simulink model "gm_sampleModel1533_sub"  (R2023a)
settings: Solver=VariableStepAuto  StartTime=0.0  StopTime=10.0  RelTol=1e-3
libraries: simulink x1
settings Model: Creator=user1  LastModifiedBy=user1
settings OptimizationCC: BlockReduction=off  ConditionallyExecuteInputs=off
settings DebuggingCC: InheritedTsInSrcMsg=none

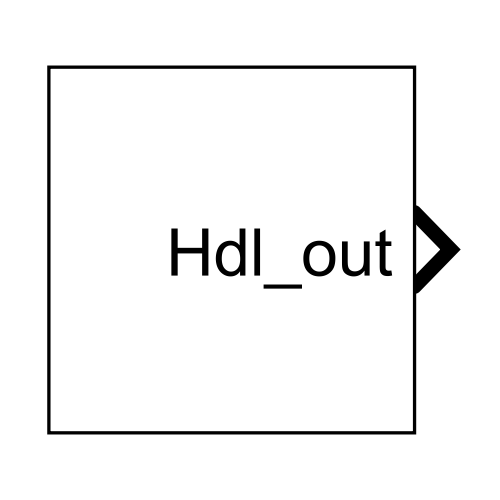
[thumbnail: Simulink's stored preview of the top-level diagram]
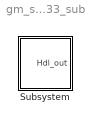
== system gm_sampleModel1533_sub ==
  Subsystem : Subsystem

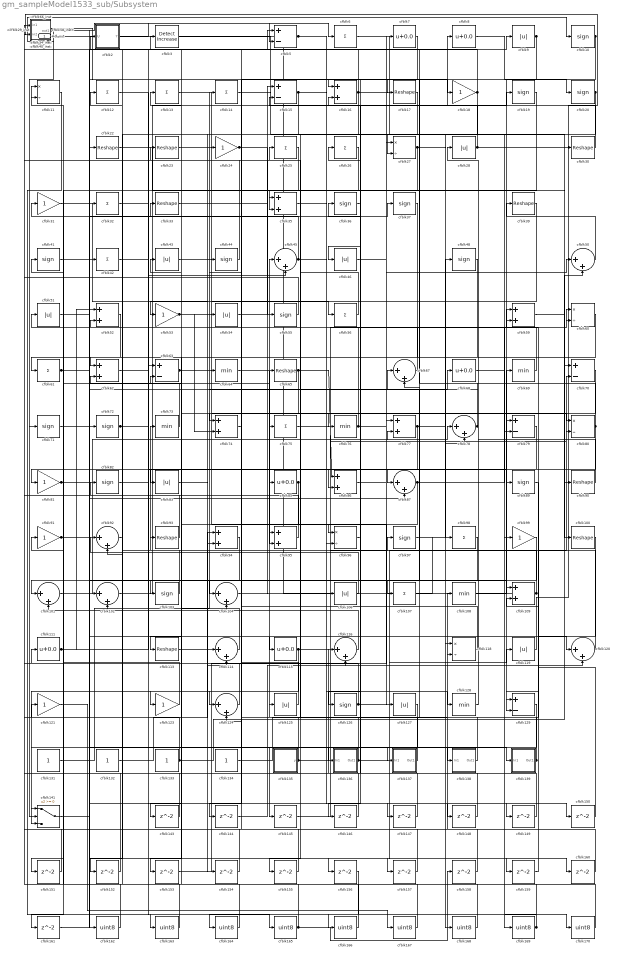
== system gm_sampleModel1533_sub/Subsystem ==
  cfblk1 : Constant  Value=0  OutDataTypeStr=uint8  SampleTime=1
  cfblk{10,19..20,36..37,41,44,48,55,71..72,82,89,97,103,126} (16 alike) : Signum
  cfblk{17,22..23,30,33,39,65,90,93,100,113} (11 alike) : Reshape
  cfblk{45,50,67,78,87,92,101..102,104,114,116,120,124} (13 alike) : Sum  Inputs=|++  OutDataTypeStr=uint8
  cfblk105_inst : Subsystem
  cfblk{9,28,43,46,51,54,83,106,119,125,127} (11 alike) : Abs  OutDataTypeStr=uint8  SaturateOnIntegerOverflow=off
  cfblk{6,12..14,25..26,32,42,56,61,75,98,107} (13 alike) : Sum  Inputs=+  OutDataTypeStr=uint8
  cfblk{64,69,73,76,108,128} (6 alike) : MinMax  OutDataTypeStr=uint8
  cfblk{16,35,52,59,62,74,77,86,94..95,109} (11 alike) : Sum  OutDataTypeStr=uint8
  cfblk{11,27,60,80,96,118} (6 alike) : Product  Inputs=*/  OutDataTypeStr=uint8  RndMeth=Zero  SaturateOnIntegerOverflow=on
  cfblk110_inst : Subsystem
  cfblk{7..8,68,85,111,115} (6 alike) : Bias  Bias=0.0  SaturateOnIntegerOverflow=off
  cfblk112_inst : Subsystem
  cfblk117_inst : Subsystem
  cfblk{18,24,31,53,81,91,99,121,123} (9 alike) : Gain  OutDataTypeStr=uint8
  cfblk122_inst : Subsystem
  cfblk{5,15,63,70,79,129} (6 alike) : Sum  Inputs=+-  OutDataTypeStr=uint8
  cfblk{131..134} (4 alike) : Constant  OutDataTypeStr=uint8  SampleTime=-1
  cfblk135 : Subsystem  mask(Counter Free-Running){NumBits=double(16), tsamp=double(-1)}
      mask prompts: NumBits "Simulink:masks:NumberOfBits_MP"; tsamp "Simulink:masks:SampleTime_MP"
      mask help: Simulink:masks:CounterFreeRunning_MD
  cfblk136 : Subsystem
  cfblk137 : Subsystem
  cfblk138 : Subsystem
  cfblk139 : Subsystem
  cfblk141 : Switch  OutDataTypeStr=uint8  SaturateOnIntegerOverflow=off  InputSameDT=off
  cfblk{143..161} (19 alike) : Delay  SampleTime=1
  cfblk{162..170} (9 alike) : DataTypeConversion  OutDataTypeStr=uint8  SaturateOnIntegerOverflow=off  RndMeth=Floor
  cfblk2 : Subsystem  mask(Detect Rise Nonnegative){vinit=double(0), InputProcessing=Elements as channels (sample based), OutDataTypeStr=uint8}
      mask prompts: vinit "Simulink:masks:InitialCondition_MP"; InputProcessing "Simulink:masks:InputProcessing_MP"; OutDataTypeStr "Simulink:masks:OutputDataType_MP"
      mask help: Simulink:masks:DetectRiseNonnegative_MD
      mask init:
      | InputProcessing = 'Elements as channels (sample based)';
      | OutDataTypeStr = 'uint8';
      | vinit = double(0);
      mask TypeOptions InputProcessing: Simulink:masks:ColumnsAsChannelsFrameBased | Simulink:masks:ElementsAsChannelsSampleBased
      mask TypeOptions OutDataTypeStr: Simulink:masks:uint8 | Simulink:masks:boolean
      mask Display: fprintf('U >= 0\n&  NOT\nU/z >= 0')
  cfblk21_inst : Subsystem
  cfblk29_inst : Subsystem
  cfblk3 : simulink/Logic and Bit Operations/Detect Increase  vinit=0.0  OutDataTypeStr=uint8
      settings: LibrarySourceBlock=|
      | hdlsllib/Logic and Bit
      | Operations/Detect
      | Increase
  cfblk34_inst : Subsystem
  cfblk40_inst : Subsystem
  cfblk58_inst : Subsystem
  cfblk66_inst : Subsystem
  Hdl_out : Outport  OutDataTypeStr=uint8  SampleTime=1
  wires:
  cfblk1/1 -> cfblk16/1
  cfblk10/1 -> cfblk67/2, cfblk46/1, cfblk129/2
  cfblk100/1 -> cfblk111/1
  cfblk101/1 -> cfblk78/1
  cfblk102/1 -> cfblk19/1
  cfblk103/1 -> cfblk73/1
  cfblk104/1 -> cfblk97/1
  cfblk105_inst/1(out1) -> cfblk10/1
  cfblk106/1 -> cfblk92/1
  cfblk107/1 -> cfblk98/1
  cfblk108/1 -> cfblk69/1
  cfblk109/1 -> Hdl_out/1, cfblk2/1(U)
  cfblk11/1 -> cfblk163/1
  cfblk110_inst/1(out1) -> cfblk22/1, cfblk160/1
  cfblk111/1 -> cfblk63/1, cfblk52/1
  cfblk112_inst/1(out1) -> cfblk109/1
  cfblk113/1 -> cfblk114/1
  cfblk114/1 -> cfblk13/1
  cfblk115/1 -> cfblk79/1, cfblk77/2, cfblk141/3
  cfblk116/1 -> cfblk101/2
  cfblk117_inst/1(out1) -> cfblk103/1
  cfblk118/1 -> cfblk33/1
  cfblk119/1 -> cfblk66_inst/2(in2)
  cfblk12/1 -> cfblk45/2
  cfblk120/1 -> cfblk59/1
  cfblk121/1 -> cfblk167/1
  cfblk122_inst/1(out1) -> cfblk162/1
  cfblk123/1 -> cfblk91/1
  cfblk124/1 -> cfblk21_inst/2(in2)
  cfblk125/1 -> cfblk93/1
  cfblk126/1 -> cfblk70/2, cfblk43/1
  cfblk127/1 -> cfblk141/1
  cfblk128/1 -> cfblk28/1
  cfblk129/1 -> cfblk145/1
  cfblk13/1 -> cfblk56/1
  cfblk131/1 -> cfblk14/1
  cfblk132/1 -> cfblk94/1
  cfblk133/1 -> cfblk62/2, cfblk50/2, cfblk112_inst/2(in2)
  cfblk134/1 -> cfblk108/1
  cfblk135/1(y) -> cfblk52/2, cfblk60/1
  cfblk136/1(Out1) -> cfblk45/1, cfblk119/1, cfblk159/1, cfblk25/1
  cfblk137/1(Out1) -> cfblk40_inst/1(in1)
  cfblk138/1(Out1) -> cfblk125/1
  cfblk139/1(Out1) -> cfblk67/1, cfblk36/1
  cfblk14/1 -> cfblk70/1
  cfblk141/1 -> cfblk72/1
  cfblk143/1 -> cfblk11/1
  cfblk144/1 -> cfblk120/2
  cfblk145/1 -> cfblk80/2
  cfblk146/1 -> cfblk105_inst/1(in1)
  cfblk147/1 -> cfblk16/2
  cfblk148/1 -> cfblk40_inst/2(in2)
  cfblk149/1 -> cfblk116/1
  cfblk15/1 -> cfblk92/2, cfblk27/2
  cfblk150/1 -> cfblk59/2
  cfblk151/1 -> cfblk117_inst/2(in2)
  cfblk152/1 -> cfblk110_inst/1(in1)
  cfblk153/1 -> cfblk77/1
  cfblk154/1 -> cfblk21_inst/1(in1)
  cfblk155/1 -> cfblk63/2
  cfblk156/1 -> cfblk164/1
  cfblk157/1 -> cfblk104/2
  cfblk158/1 -> cfblk58_inst/1(in1)
  cfblk159/1 -> cfblk109/2
  cfblk16/1 -> cfblk95/2, cfblk78/2, cfblk112_inst/1(in1)
  cfblk160/1 -> cfblk118/2
  cfblk161/1 -> cfblk9/1
  cfblk162/1 -> cfblk58_inst/2(in2)
  cfblk163/1 -> cfblk122_inst/1(in1)
  cfblk164/1 -> cfblk122_inst/2(in2)
  cfblk165/1 -> cfblk158/1, cfblk12/1
  cfblk166/1 -> cfblk82/1
  cfblk167/1 -> cfblk34_inst/1(in1)
  cfblk168/1 -> cfblk121/1
  cfblk169/1 -> cfblk34_inst/2(in2), cfblk166/1
  cfblk17/1 -> cfblk94/2
  cfblk170/1 -> cfblk3/1
  cfblk18/1 -> cfblk66_inst/1(in1), cfblk62/1
  cfblk19/1 -> cfblk35/2
  cfblk2/1(Y) -> cfblk6/1
  cfblk20/1 -> cfblk87/1, cfblk124/2
  cfblk21_inst/1(out1) -> cfblk71/1, cfblk156/1
  cfblk22/1 -> cfblk100/1
  cfblk23/1 -> cfblk127/1
  cfblk24/1 -> cfblk106/1, cfblk96/1
  cfblk25/1 -> cfblk81/1
  cfblk26/1 -> cfblk35/1
  cfblk27/1 -> cfblk168/1, cfblk146/1
  cfblk28/1 -> cfblk8/1, cfblk30/1
  cfblk29_inst/1(out1) -> cfblk141/2, cfblk18/1
  cfblk3/1 -> cfblk169/1
  cfblk30/1 -> cfblk15/2
  cfblk31/1 -> cfblk114/2
  cfblk32/1 -> cfblk136/1(In1)
  cfblk33/1 -> cfblk55/1
  cfblk34_inst/1(out1) -> cfblk5/2, cfblk116/2
  cfblk35/1 -> cfblk79/2
  cfblk36/1 -> cfblk126/1
  cfblk37/1 -> cfblk101/1
  cfblk39/1 -> cfblk53/1
  cfblk40_inst/1(out1) -> cfblk42/1
  cfblk41/1 -> cfblk32/1
  cfblk42/1 -> cfblk138/1(In1)
  cfblk43/1 -> cfblk96/2
  cfblk44/1 -> cfblk29_inst/1(in1)
  cfblk45/1 -> cfblk31/1, cfblk128/1
  cfblk46/1 -> cfblk27/1
  cfblk48/1 -> cfblk123/1
  cfblk5/1 -> cfblk148/1, cfblk147/1
  cfblk50/1 -> cfblk39/1
  cfblk51/1 -> cfblk150/1
  cfblk52/1 -> cfblk61/1
  cfblk53/1 -> cfblk89/1, cfblk74/2
  cfblk54/1 -> cfblk15/1
  cfblk55/1 -> cfblk117_inst/1(in1)
  cfblk56/1 -> cfblk23/1
  cfblk58_inst/1(out1) -> cfblk120/1
  cfblk59/1 -> cfblk90/1
  cfblk6/1 -> cfblk118/1
  cfblk60/1 -> cfblk83/1
  cfblk61/1 -> cfblk115/1, cfblk137/1(In1)
  cfblk62/1 -> cfblk86/2
  cfblk63/1 -> cfblk95/1, cfblk99/1
  cfblk64/1 -> cfblk75/1
  cfblk65/1 -> cfblk86/1, cfblk104/1
  cfblk66_inst/1(out1) -> cfblk102/1
  cfblk67/1 -> cfblk54/1
  cfblk68/1 -> cfblk170/1
  cfblk69/1 -> cfblk44/1
  cfblk7/1 -> cfblk17/1
  cfblk70/1 -> cfblk153/1
  cfblk71/1 -> cfblk87/2
  cfblk72/1 -> cfblk5/1, cfblk149/1
  cfblk73/1 -> cfblk11/2
  cfblk74/1 -> cfblk24/1
  cfblk75/1 -> cfblk80/1
  cfblk76/1 -> cfblk7/1, cfblk51/1
  cfblk77/1 -> cfblk102/2, cfblk139/1(In1)
  cfblk78/1 -> cfblk29_inst/2(in2), cfblk76/1
  cfblk79/1 -> cfblk151/1
  cfblk8/1 -> cfblk20/1
  cfblk80/1 -> cfblk85/1, cfblk110_inst/2(in2)
  cfblk81/1 -> cfblk68/1, cfblk65/1
  cfblk82/1 -> cfblk165/1
  cfblk83/1 -> cfblk154/1
  cfblk85/1 -> cfblk144/1, cfblk143/1
  cfblk86/1 -> cfblk50/1
  cfblk87/1 -> cfblk60/2, cfblk155/1
  cfblk89/1 -> cfblk129/1
  cfblk9/1 -> cfblk74/1, cfblk107/1
  cfblk90/1 -> cfblk64/1
  cfblk91/1 -> cfblk37/1, cfblk157/1
  cfblk92/1 -> cfblk152/1
  cfblk93/1 -> cfblk105_inst/2(in2)
  cfblk94/1 -> cfblk113/1
  cfblk95/1 -> cfblk41/1
  cfblk96/1 -> cfblk26/1
  cfblk97/1 -> cfblk48/1
  cfblk98/1 -> cfblk161/1
  cfblk99/1 -> cfblk124/1

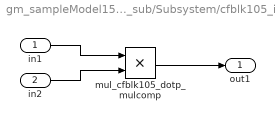
== system gm_sampleModel1533_sub/Subsystem/cfblk105_inst ==
  in1 : Inport  OutDataTypeStr=uint8  SampleTime=1
  in2 : Inport  Port=2  OutDataTypeStr=uint8  SampleTime=1
  mul_cfblk105_dotp_mulcomp : Product  Inputs=**  OutDataTypeStr=uint8  SampleTime=1
  out1 : Outport  OutDataTypeStr=uint8  SampleTime=1
  wires:
  in1/1 -> mul_cfblk105_dotp_mulcomp/1
  in2/1 -> mul_cfblk105_dotp_mulcomp/2
  mul_cfblk105_dotp_mulcomp/1 -> out1/1

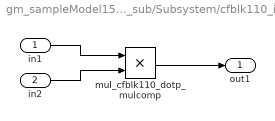
== system gm_sampleModel1533_sub/Subsystem/cfblk110_inst ==
  in1 : Inport  OutDataTypeStr=uint8  SampleTime=1
  in2 : Inport  Port=2  OutDataTypeStr=uint8  SampleTime=1
  mul_cfblk110_dotp_mulcomp : Product  Inputs=**  OutDataTypeStr=uint8  SampleTime=1
  out1 : Outport  OutDataTypeStr=uint8  SampleTime=1
  wires:
  in1/1 -> mul_cfblk110_dotp_mulcomp/1
  in2/1 -> mul_cfblk110_dotp_mulcomp/2
  mul_cfblk110_dotp_mulcomp/1 -> out1/1

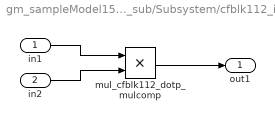
== system gm_sampleModel1533_sub/Subsystem/cfblk112_inst ==
  in1 : Inport  OutDataTypeStr=uint8  SampleTime=1
  in2 : Inport  Port=2  OutDataTypeStr=uint8  SampleTime=1
  mul_cfblk112_dotp_mulcomp : Product  Inputs=**  OutDataTypeStr=uint8  SampleTime=1
  out1 : Outport  OutDataTypeStr=uint8  SampleTime=1
  wires:
  in1/1 -> mul_cfblk112_dotp_mulcomp/1
  in2/1 -> mul_cfblk112_dotp_mulcomp/2
  mul_cfblk112_dotp_mulcomp/1 -> out1/1

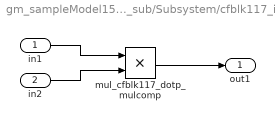
== system gm_sampleModel1533_sub/Subsystem/cfblk117_inst ==
  in1 : Inport  OutDataTypeStr=uint8  SampleTime=1
  in2 : Inport  Port=2  OutDataTypeStr=uint8  SampleTime=1
  mul_cfblk117_dotp_mulcomp : Product  Inputs=**  OutDataTypeStr=uint8  SampleTime=1
  out1 : Outport  OutDataTypeStr=uint8  SampleTime=1
  wires:
  in1/1 -> mul_cfblk117_dotp_mulcomp/1
  in2/1 -> mul_cfblk117_dotp_mulcomp/2
  mul_cfblk117_dotp_mulcomp/1 -> out1/1

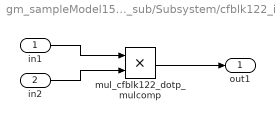
== system gm_sampleModel1533_sub/Subsystem/cfblk122_inst ==
  in1 : Inport  OutDataTypeStr=uint8  SampleTime=1
  in2 : Inport  Port=2  OutDataTypeStr=uint8  SampleTime=1
  mul_cfblk122_dotp_mulcomp : Product  Inputs=**  OutDataTypeStr=uint8  SampleTime=1
  out1 : Outport  OutDataTypeStr=uint8  SampleTime=1
  wires:
  in1/1 -> mul_cfblk122_dotp_mulcomp/1
  in2/1 -> mul_cfblk122_dotp_mulcomp/2
  mul_cfblk122_dotp_mulcomp/1 -> out1/1

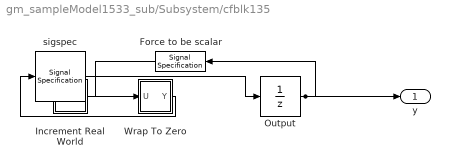
== system gm_sampleModel1533_sub/Subsystem/cfblk135 ==
  Force to be scalar : SignalSpecification  DisableCoverage=on  Dimensions=1
  Increment Real World : Subsystem  mask(Real World Value Increment){}
      mask help: Simulink:masks:RealWorldValueIncrement_MD
      mask Display: disp('V++')
  Output : UnitDelay  InitialCondition=0.0  SampleTime=tsamp  HasFrameUpgradeWarning=on
  Wrap To Zero : Subsystem  mask(Wrap To Zero){Threshold=double(65535)}
      mask prompts: Threshold "Simulink:masks:Threshold_MP"
      mask help: Simulink:masks:WrapToZero_MD
  sigspec : SignalSpecification  OutDataTypeStr=uint16  Dimensions=1
  y : Outport  SampleTime=1
  wires:
  Force to be scalar/1 -> Increment Real World/1(u)
  Increment Real World/1(y) -> Wrap To Zero/1(U)
  Output/1 -> Force to be scalar/1, y/1
  Wrap To Zero/1(Y) -> sigspec/1
  sigspec/1 -> Output/1

== system gm_sampleModel1533_sub/Subsystem/cfblk136 ==
  In1 : Inport  OutDataTypeStr=uint8  PortDimensions=1  SampleTime=1
  Out1 : Outport  SampleTime=1
  wires:
  In1/1 -> Out1/1

== system gm_sampleModel1533_sub/Subsystem/cfblk137 ==
  In1 : Inport  OutDataTypeStr=uint8  PortDimensions=1  SampleTime=1
  Out1 : Outport  SampleTime=1
  wires:
  In1/1 -> Out1/1

== system gm_sampleModel1533_sub/Subsystem/cfblk138 ==
  In1 : Inport  OutDataTypeStr=uint8  PortDimensions=1  SampleTime=1
  Out1 : Outport  SampleTime=1
  wires:
  In1/1 -> Out1/1

== system gm_sampleModel1533_sub/Subsystem/cfblk139 ==
  In1 : Inport  OutDataTypeStr=uint8  PortDimensions=1  SampleTime=1
  Out1 : Outport  SampleTime=1
  wires:
  In1/1 -> Out1/1

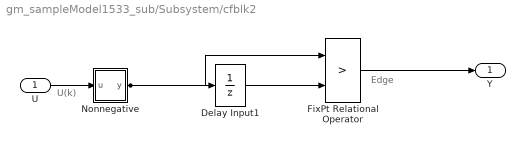
== system gm_sampleModel1533_sub/Subsystem/cfblk2 ==
  note: U(k)
  note: Edge
  U : Inport  OutDataTypeStr=uint8  SampleTime=1
  Delay Input1 : UnitDelay  Description=Store in Global RAM  DisableCoverage=on  InitialCondition=vinit  SampleTime=-1  HasFrameUpgradeWarning=on
  FixPt Relational Operator : RelationalOperator  Operator=>  OutDataTypeStr=fixdt(0, 8)  ZeroCross=off  InputSameDT=off
  Nonnegative : Subsystem  mask(Compare To Zero){relop=>=, OutDataTypeStr=boolean, ZeroCross=off}
      mask prompts: relop "Simulink:masks:Operator_MP"; OutDataTypeStr "Simulink:masks:OutputDataType_MP"; ZeroCross "Simulink:masks:EnableZerocrossingDetection_MP"
      mask help: Simulink:masks:CompareToZero_MD
      mask init:
      | OutDataTypeStr = 'boolean';
      | ZeroCross = 'off';
      | blkName = 'sampleModel1533_sub/Subsystem/cfblk2/Nonnegative';
      | relop = '>=';
      | setValue = 'boolean';
      mask TypeOptions relop: == | ~= | < | <= | >= | >
      mask TypeOptions OutDataTypeStr: Simulink:masks:uint8 | Simulink:masks:boolean
      mask Callback ZeroCross: sl('zeroCrossEnable', gcbh);
      mask Display: disp([relop,' 0'])
  Y : Outport  SampleTime=1
  wires:
  U/1 -> Nonnegative/1(u)
  Delay Input1/1 -> FixPt Relational Operator/2
  FixPt Relational Operator/1 -> Y/1
  Nonnegative/1(y) -> FixPt Relational Operator/1, Delay Input1/1

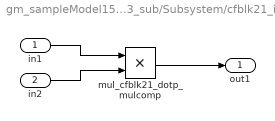
== system gm_sampleModel1533_sub/Subsystem/cfblk21_inst ==
  in1 : Inport  OutDataTypeStr=uint8  SampleTime=1
  in2 : Inport  Port=2  OutDataTypeStr=uint8  SampleTime=1
  mul_cfblk21_dotp_mulcomp : Product  Inputs=**  OutDataTypeStr=uint8  SampleTime=1
  out1 : Outport  OutDataTypeStr=uint8  SampleTime=1
  wires:
  in1/1 -> mul_cfblk21_dotp_mulcomp/1
  in2/1 -> mul_cfblk21_dotp_mulcomp/2
  mul_cfblk21_dotp_mulcomp/1 -> out1/1

== system gm_sampleModel1533_sub/Subsystem/cfblk29_inst ==
  in1 : Inport  OutDataTypeStr=uint8  SampleTime=1
  in2 : Inport  Port=2  OutDataTypeStr=uint8  SampleTime=1
  mul_cfblk29_dotp_mulcomp : Product  Inputs=**  OutDataTypeStr=uint8  SampleTime=1
  out1 : Outport  OutDataTypeStr=uint8  SampleTime=1
  wires:
  in1/1 -> mul_cfblk29_dotp_mulcomp/1
  in2/1 -> mul_cfblk29_dotp_mulcomp/2
  mul_cfblk29_dotp_mulcomp/1 -> out1/1

== system gm_sampleModel1533_sub/Subsystem/cfblk34_inst ==
  in1 : Inport  OutDataTypeStr=uint8  SampleTime=1
  in2 : Inport  Port=2  OutDataTypeStr=uint8  SampleTime=1
  mul_cfblk34_dotp_mulcomp : Product  Inputs=**  OutDataTypeStr=uint8  SampleTime=1
  out1 : Outport  OutDataTypeStr=uint8  SampleTime=1
  wires:
  in1/1 -> mul_cfblk34_dotp_mulcomp/1
  in2/1 -> mul_cfblk34_dotp_mulcomp/2
  mul_cfblk34_dotp_mulcomp/1 -> out1/1

== system gm_sampleModel1533_sub/Subsystem/cfblk40_inst ==
  in1 : Inport  OutDataTypeStr=uint8  SampleTime=1
  in2 : Inport  Port=2  OutDataTypeStr=uint8  SampleTime=1
  mul_cfblk40_dotp_mulcomp : Product  Inputs=**  OutDataTypeStr=uint8  SampleTime=1
  out1 : Outport  OutDataTypeStr=uint8  SampleTime=1
  wires:
  in1/1 -> mul_cfblk40_dotp_mulcomp/1
  in2/1 -> mul_cfblk40_dotp_mulcomp/2
  mul_cfblk40_dotp_mulcomp/1 -> out1/1

== system gm_sampleModel1533_sub/Subsystem/cfblk58_inst ==
  in1 : Inport  OutDataTypeStr=uint8  SampleTime=1
  in2 : Inport  Port=2  OutDataTypeStr=uint8  SampleTime=1
  mul_cfblk58_dotp_mulcomp : Product  Inputs=**  OutDataTypeStr=uint8  SampleTime=1
  out1 : Outport  OutDataTypeStr=uint8  SampleTime=1
  wires:
  in1/1 -> mul_cfblk58_dotp_mulcomp/1
  in2/1 -> mul_cfblk58_dotp_mulcomp/2
  mul_cfblk58_dotp_mulcomp/1 -> out1/1

== system gm_sampleModel1533_sub/Subsystem/cfblk66_inst ==
  in1 : Inport  OutDataTypeStr=uint8  SampleTime=1
  in2 : Inport  Port=2  OutDataTypeStr=uint8  SampleTime=1
  mul_cfblk66_dotp_mulcomp : Product  Inputs=**  OutDataTypeStr=uint8  SampleTime=1
  out1 : Outport  OutDataTypeStr=uint8  SampleTime=1
  wires:
  in1/1 -> mul_cfblk66_dotp_mulcomp/1
  in2/1 -> mul_cfblk66_dotp_mulcomp/2
  mul_cfblk66_dotp_mulcomp/1 -> out1/1

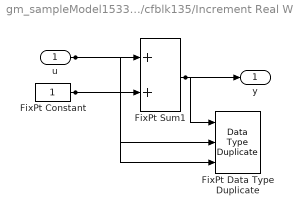
== system gm_sampleModel1533_sub/Subsystem/cfblk135/Increment Real World ==
  u : Inport  OutDataTypeStr=uint16  SampleTime=1
  FixPt Constant : Constant  DisableCoverage=on  OutDataTypeStr=Inherit: Inherit via back propagation  SampleTime=-1
  FixPt Data Type Duplicate : DataTypeDuplicate  DisableCoverage=on  NumInputPorts=3
  FixPt Sum1 : Sum  InputSameDT=on  OutDataTypeStr=Inherit: Inherit via back propagation  LockScale=on
  y : Outport  SampleTime=1
  wires:
  u/1 -> FixPt Sum1/1, FixPt Data Type Duplicate/2
  FixPt Constant/1 -> FixPt Sum1/2, FixPt Data Type Duplicate/3
  FixPt Sum1/1 -> FixPt Data Type Duplicate/1, y/1

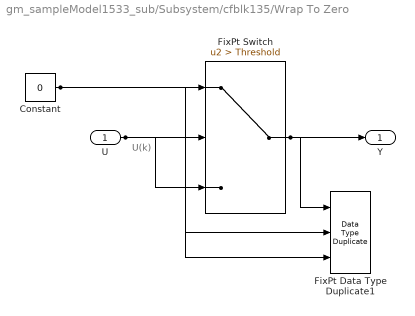
== system gm_sampleModel1533_sub/Subsystem/cfblk135/Wrap To Zero ==
  note: U(k)
  U : Inport  OutDataTypeStr=uint16  SampleTime=1
  Constant : Constant  DisableCoverage=on  Value=0  OutDataTypeStr=Inherit: Inherit via back propagation  SampleTime=-1
  FixPt Data Type Duplicate1 : DataTypeDuplicate  DisableCoverage=on  NumInputPorts=3
  FixPt Switch : Switch  Criteria=u2 > Threshold  Threshold=Threshold  OutDataTypeStr=Inherit: Inherit via back propagation  ZeroCross=off  SaturateOnIntegerOverflow=off  InputSameDT=off
  Y : Outport  SampleTime=1
  wires:
  U/1 -> FixPt Switch/3, FixPt Switch/2, FixPt Data Type Duplicate1/2
  Constant/1 -> FixPt Switch/1, FixPt Data Type Duplicate1/3
  FixPt Switch/1 -> FixPt Data Type Duplicate1/1, Y/1

== system gm_sampleModel1533_sub/Subsystem/cfblk2/Nonnegative ==
  u : Inport  OutDataTypeStr=uint8  SampleTime=1
  Compare : RelationalOperator  OutDataTypeStr=boolean  ZeroCross=off
  Constant : Constant  DisableCoverage=on  Value=0  OutDataTypeStr=Inherit: Inherit via back propagation  SampleTime=-1  PreserveConstantTs=on
  y : Outport  SampleTime=1
  wires:
  u/1 -> Compare/1
  Compare/1 -> y/1
  Constant/1 -> Compare/2
